simulink model "dcpController_ExperimentalPosVel"  (R2016b)
settings: Solver=ode5  StartTime=0.0  StopTime=inf  FixedStep=0.001  RelTol=1e-3  EnableMultiTasking=on
undefined symbols (not defined in the file): robot, Standard_Devices, UDP_Protocol
libraries: dcpctrl x20, simulink x6, kukaslxctrl x1, sldrtlib x1
(part 1 of 2)
settings Model: SimulationMode=external  Creator=julianleland  LastModifiedBy=julianleland
settings OptimizationCC: LifeSpan=inf
settings DebuggingCC: SFUnexpectedBacktrackingDiag=warning  SFNoUnconditionalDefaultTransitionDiag=warning  SFExecutionAtInitializationDiag=none
settings HardwareCC: ProdBitPerLong=64  ProdHWDeviceType=Intel->x86-64 (Mac OS X)  TargetBitPerLong=64  TargetBitPerPointer=64  TargetIntDivRoundTo=Zero  TargetEndianess=LittleEndian  TargetWordSize=64  TargetHWDeviceType=Intel->x86-64
settings RTWCC: SystemTargetFile=sldrt.tlc  TemplateMakefile=sldrt.tmf  Description=Simulink Desktop Real-Time  RTWCompilerOptimization=on
settings CodeAppCC: MaxIdLength=95
settings SimulinkDesktopRealTimeCC: TargetPreCompLibLocation=/Applications/MATLAB_R2016b.app/toolbox/sldrt/lib/maci64  TargetLangStandard=C89/C90 (ANSI)  SupportVariableSizeSignals=off
settings ConfigComp: CovMetricSettings=dw  CovHtmlReporting=on  CovSaveCumulativeToWorkspaceVar=on  CovSaveSingleToWorkspaceVar=on  CovExternalEMLEnable=off

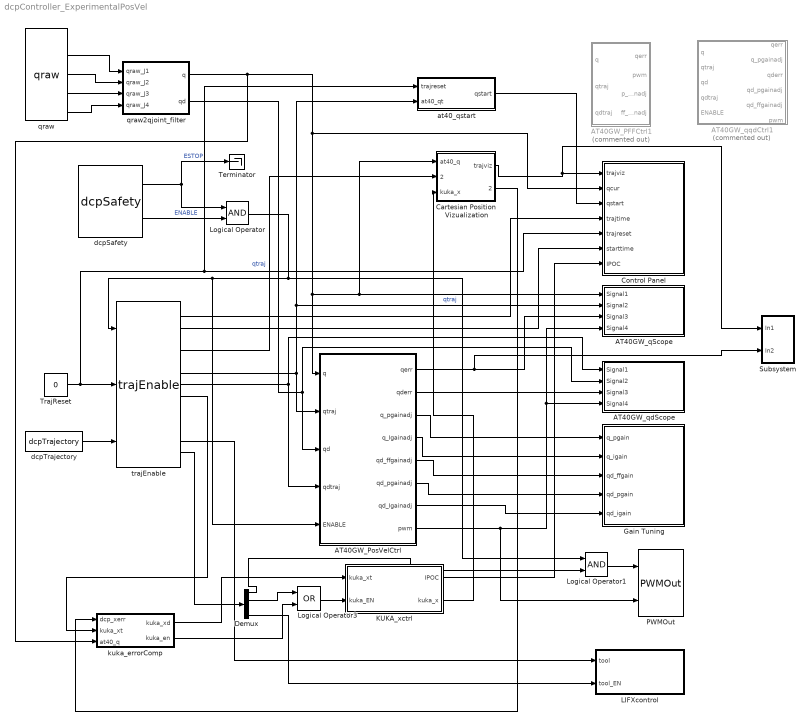
== system dcpController_ExperimentalPosVel ==
  AT40GW_PFFCtrl1 : Subsystem  Commented=on
  AT40GW_PosVelCtrl : Subsystem
  AT40GW_qScope : Subsystem  AncestorBlock=dcpctrl/AT40GW_qScope
  AT40GW_qdScope : Subsystem  AncestorBlock=dcpctrl/AT40GW_qScope
  AT40GW_qqdCtrl1 : Subsystem  Commented=on
  Cartesian Position Vizualization : Subsystem
  Control Panel : Subsystem
  Demux : Demux
  Gain Tuning : Subsystem
  KUKA_xctrl : Subsystem
  LIFXcontrol : Subsystem
  Logical Operator : Logic  AllPortsSameDT=off  OutDataTypeStr=boolean
  Logical Operator1 : Logic  AllPortsSameDT=off  OutDataTypeStr=boolean
  Logical Operator3 : Logic  Operator=OR  AllPortsSameDT=off  OutDataTypeStr=boolean
  PWMOut : dcpctrl/PWMOut
  Subsystem : Subsystem
  Terminator : Terminator
  TrajReset : Constant  Value=0
  at40_qstart : Subsystem
  dcpSafety : dcpctrl/dcpSafety
  dcpTrajectory : dcpctrl/dcpTrajectory
  kuka_errorComp : Subsystem
  qraw : dcpctrl/qraw
  qraw2qjoint_filter : Subsystem
  trajEnable : dcpctrl/trajEnable
      link override "Stoppable Time/Trajectory Time ": Gain=0
  wires:
  trajEnable/6 -> AT40GW_PosVelCtrl/2(qtraj), at40_qstart/2(at40_qt), AT40GW_qScope/2(Signal2)  "qtraj"
  dcpSafety/1 -> Logical Operator/1, Terminator/1  "ESTOP"
  dcpSafety/2 -> Logical Operator/2  "ENABLE"
  TrajReset/1 -> at40_qstart/1(trajreset), Control Panel/5(trajreset), trajEnable/2
  trajEnable/1 -> Control Panel/4(trajtime)
  qraw2qjoint_filter/1(q) -> kuka_errorComp/3(at40_q), AT40GW_PosVelCtrl/1(q), Cartesian Position Vizualization/1(at40_q), AT40GW_qScope/1(Signal1), Control Panel/2(qcur)
  trajEnable/12 -> LIFXcontrol/1(tool)
  dcpTrajectory/1 -> trajEnable/3
  trajEnable/2 -> Control Panel/6(starttime)
  qraw/2 -> qraw2qjoint_filter/1(qraw_J1)
  qraw/3 -> qraw2qjoint_filter/2(qraw_J2)
  qraw/4 -> qraw2qjoint_filter/3(qraw_J3)
  qraw/5 -> qraw2qjoint_filter/4(qraw_J4)
  Cartesian Position Vizualization/1(trajviz) -> Subsystem/1(In1), Control Panel/1(trajviz)
  KUKA_xctrl/1(IPOC) -> Control Panel/7(IPOC)
  trajEnable/8 -> kuka_errorComp/2("kuka_xt ")
  trajEnable/13 -> Demux/1
  Demux/4 -> LIFXcontrol/2(tool_EN)
  Logical Operator1/1 -> PWMOut/1
  Demux/1 -> Logical Operator1/2
  KUKA_xctrl/2(kuka_x) -> Cartesian Position Vizualization/3(kuka_x)
  trajEnable/4 -> Cartesian Position Vizualization/2(dcp_xdes)  "qtraj"
  qraw2qjoint_filter/2(qd) -> AT40GW_PosVelCtrl/3(qd), AT40GW_qdScope/2(Signal2)
  Logical Operator/1 -> Logical Operator1/1, AT40GW_PosVelCtrl/5(ENABLE), trajEnable/1
  AT40GW_PosVelCtrl/2(qderr) -> AT40GW_qdScope/3(Signal3)
  AT40GW_PosVelCtrl/8(pwm) -> AT40GW_qdScope/4(Signal4), AT40GW_qScope/4(Signal4), PWMOut/2
  trajEnable/7 -> AT40GW_qdScope/1(Signal1), AT40GW_PosVelCtrl/4(qdtraj)
  AT40GW_PosVelCtrl/1(qerr) -> Subsystem/2(In2), AT40GW_qScope/3(Signal3)
  AT40GW_PosVelCtrl/3(q_pgainadj) -> Gain Tuning/1(q_pgain)
  AT40GW_PosVelCtrl/5(qd_ffgainadj) -> Gain Tuning/3(qd_ffgain)
  AT40GW_PosVelCtrl/6(qd_pgainadj) -> Gain Tuning/4(qd_pgain)
  AT40GW_PosVelCtrl/4(q_Igainadj) -> Gain Tuning/2(q_igain)
  AT40GW_PosVelCtrl/7(qd_Igainadj) -> Gain Tuning/5(qd_igain)
  kuka_errorComp/1(kuka_xd) -> KUKA_xctrl/1("kuka_xt   ")
  Cartesian Position Vizualization/2(dcp_xerr) -> kuka_errorComp/1(dcp_xerr)
  Logical Operator3/1 -> KUKA_xctrl/2(kuka_EN)
  Demux/2 -> Logical Operator3/1
  kuka_errorComp/2(kuka_en) -> Logical Operator3/2
  at40_qstart/1(qstart) -> Control Panel/3(qstart)

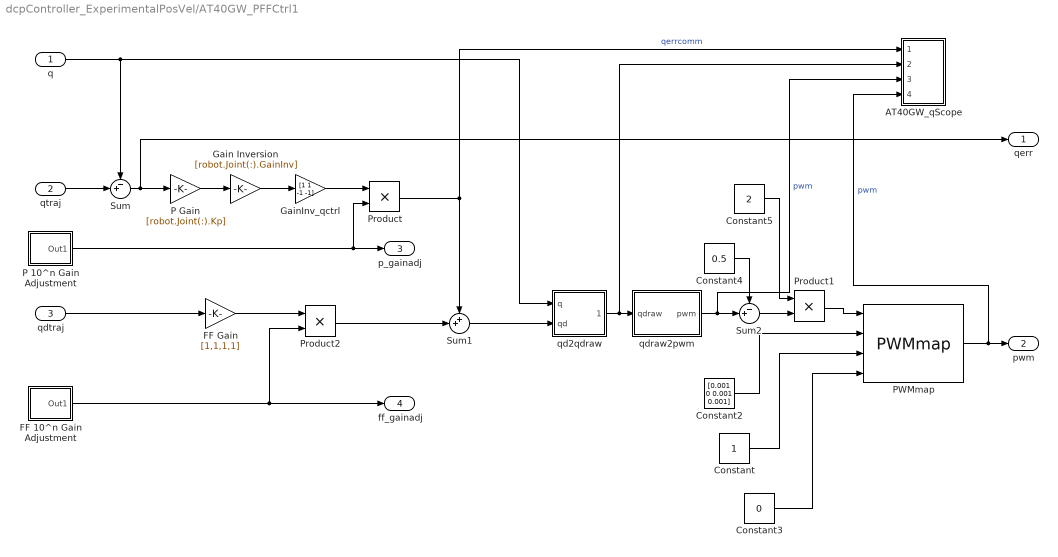
== system dcpController_ExperimentalPosVel/AT40GW_PFFCtrl1 ==
  q : Inport
  qtraj : Inport  Port=2
  qdtraj : Inport  Port=3
  AT40GW_qScope : Subsystem
  Constant : Constant
  Constant2 : Constant  Value=[0.001 0 0.001 0.001]
  Constant3 : Constant  Value=0
  Constant4 : Constant  Value=0.5
  Constant5 : Constant  Value=2
  FF 10^n Gain Adjustment : Subsystem
  FF Gain : Gain  Gain=[1,1,1,1]
  Gain Inversion : Gain  Gain=[robot.Joint(:).GainInv]
  GainInv_qctrl : Gain  Gain=[1 1 -1 -1]
  P 10^n Gain Adjustment : Subsystem
  P Gain : Gain  Gain=[robot.Joint(:).Kp]
  PWMmap : dcpctrl/PWMmap
  Product : Product
  Product1 : Product
  Product2 : Product
  Sum : Sum  Inputs=-+|
  Sum1 : Sum  Inputs=++|
  Sum2 : Sum  Inputs=-+|
  qd2qdraw : Subsystem
  qdraw2pwm : Subsystem
  qerr : Outport
  pwm : Outport  Port=2
  p_gainadj : Outport  Port=3
  ff_gainadj : Outport  Port=4
  wires:
  Product2/1 -> Sum1/2
  FF 10^n Gain Adjustment/1(Out1) -> Product2/2, ff_gainadj/1
  P 10^n Gain Adjustment/1(Out1) -> Product/2, p_gainadj/1
  Product/1 -> AT40GW_qScope/1(Signal1), Sum1/1  "qerrcomm"
  PWMmap/1 -> pwm/1, AT40GW_qScope/4(Signal4)  "pwm"
  FF Gain/1 -> Product2/1
  qdtraj/1 -> FF Gain/1
  Constant5/1 -> Product1/1
  Product1/1 -> PWMmap/1
  Sum2/1 -> Product1/2
  Constant4/1 -> Sum2/1
  qdraw2pwm/1(pwm) -> Sum2/2, AT40GW_qScope/3(Signal3)  "pwm"
  GainInv_qctrl/1 -> Product/1
  qd2qdraw/1(qdraw) -> qdraw2pwm/1(qdraw), AT40GW_qScope/2(Signal2)
  q/1 -> Sum/1, qd2qdraw/1(q)
  Sum1/1 -> qd2qdraw/2(qd)
  Gain Inversion/1 -> GainInv_qctrl/1
  Constant2/1 -> PWMmap/2
  Constant3/1 -> PWMmap/4
  Constant/1 -> PWMmap/3
  P Gain/1 -> Gain Inversion/1
  Sum/1 -> qerr/1, P Gain/1
  qtraj/1 -> Sum/2

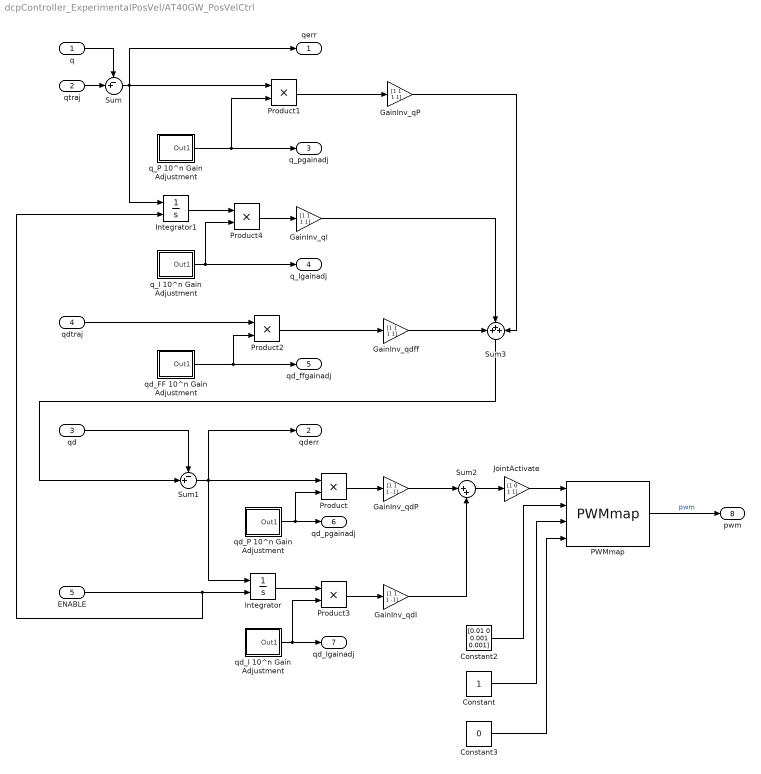
== system dcpController_ExperimentalPosVel/AT40GW_PosVelCtrl ==
  q : Inport
  qtraj : Inport  Port=2
  qd : Inport  Port=3
  qdtraj : Inport  Port=4
  ENABLE : Inport  Port=5
  Constant : Constant
  Constant2 : Constant  Value=[0.01 0 0.001 0.001]
  Constant3 : Constant  Value=0
  GainInv_qI : Gain  Gain=[1 1 1 1]
  GainInv_qP : Gain  Gain=[1 1 1 1]
  GainInv_qdI : Gain  Gain=[1 1 1 -1]
  GainInv_qdP : Gain  Gain=[1 1 1 -1]
  GainInv_qdff : Gain  Gain=[1 1 1 1]
  Integrator : Integrator  ExternalReset=rising  LimitOutput=on  UpperSaturationLimit=[100 10 100 1000]  LowerSaturationLimit=[-100 -10 -100 -1000]
  Integrator1 : Integrator  ExternalReset=rising  LimitOutput=on  UpperSaturationLimit=[10 2 10 20]  LowerSaturationLimit=[-10 -2 -10 -20]
  JointActivate : Gain  Gain=[1 0 1 1]
  PWMmap : dcpctrl/PWMmap
  Product{,1..4} (5 alike) : Product
  Sum : Sum  Inputs=-+|
  Sum1 : Sum  Inputs=-+|
  Sum2 : Sum  Inputs=|++
  Sum3 : Sum  Inputs=+++
  q_I 10^n Gain Adjustment : Subsystem
  q_P 10^n Gain Adjustment : Subsystem
  qd_FF 10^n Gain Adjustment : Subsystem
  qd_I 10^n Gain Adjustment : Subsystem
  qd_P 10^n Gain Adjustment : Subsystem
  qerr : Outport
  qderr : Outport  Port=2
  q_pgainadj : Outport  Port=3
  q_Igainadj : Outport  Port=4
  qd_ffgainadj : Outport  Port=5
  qd_pgainadj : Outport  Port=6
  qd_Igainadj : Outport  Port=7
  pwm : Outport  Port=8
  wires:
  GainInv_qdff/1 -> Sum3/1
  Sum3/1 -> Sum1/2
  GainInv_qdI/1 -> Sum2/2
  ENABLE/1 -> Integrator/2, Integrator1/2
  Integrator1/1 -> Product4/1
  Product4/1 -> GainInv_qI/1
  q_I 10^n Gain Adjustment/1(Out1) -> q_Igainadj/1, Product4/2
  Sum/1 -> Integrator1/1, qerr/1, Product1/1
  Sum2/1 -> JointActivate/1
  qdtraj/1 -> Product2/1
  qd/1 -> Sum1/1
  Integrator/1 -> Product3/1
  GainInv_qdP/1 -> Sum2/1
  Product3/1 -> GainInv_qdI/1
  qd_I 10^n Gain Adjustment/1(Out1) -> qd_Igainadj/1, Product3/2
  q_P 10^n Gain Adjustment/1(Out1) -> Product1/2, q_pgainadj/1
  Product/1 -> GainInv_qdP/1
  q/1 -> Sum/1
  Product2/1 -> GainInv_qdff/1
  Sum1/1 -> qderr/1, Product/1, Integrator/1
  qd_FF 10^n Gain Adjustment/1(Out1) -> Product2/2, qd_ffgainadj/1
  qd_P 10^n Gain Adjustment/1(Out1) -> Product/2, qd_pgainadj/1
  PWMmap/1 -> pwm/1  "pwm"
  Product1/1 -> GainInv_qP/1
  Constant2/1 -> PWMmap/2
  Constant3/1 -> PWMmap/4
  Constant/1 -> PWMmap/3
  qtraj/1 -> Sum/2
  JointActivate/1 -> PWMmap/1
  GainInv_qI/1 -> Sum3/2
  GainInv_qP/1 -> Sum3/3

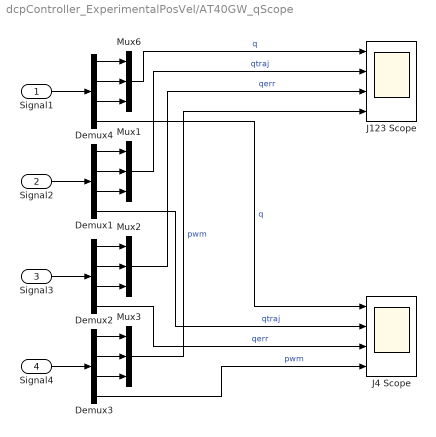
== system dcpController_ExperimentalPosVel/AT40GW_qScope ==
  Signal1 : Inport
  Signal2 : Inport  Port=2
  Signal3 : Inport  Port=3
  Signal4 : Inport  Port=4
  Demux{1..4} (4 alike) : Demux
  J123 Scope : Scope  NumInputPorts=4
  J4 Scope : Scope  NumInputPorts=4
  Mux{1..3,6} (4 alike) : Mux  Inputs=3
  wires:
  Demux4/1 -> Mux6/1
  Mux3/1 -> J123 Scope/4  "pwm"
  Demux2/4 -> J4 Scope/3  "qerr"
  Demux1/4 -> J4 Scope/2  "qtraj"
  Mux6/1 -> J123 Scope/1  "q"
  Signal1/1 -> Demux4/1
  Demux4/2 -> Mux6/2
  Demux4/3 -> Mux6/3
  Demux1/1 -> Mux1/1
  Signal2/1 -> Demux1/1
  Demux1/2 -> Mux1/2
  Demux1/3 -> Mux1/3
  Demux2/1 -> Mux2/1
  Signal3/1 -> Demux2/1
  Demux2/2 -> Mux2/2
  Demux2/3 -> Mux2/3
  Demux3/1 -> Mux3/1
  Signal4/1 -> Demux3/1
  Demux3/2 -> Mux3/2
  Demux3/3 -> Mux3/3
  Mux1/1 -> J123 Scope/2  "qtraj"
  Mux2/1 -> J123 Scope/3  "qerr"
  Demux4/4 -> J4 Scope/1  "q"
  Demux3/4 -> J4 Scope/4  "pwm"

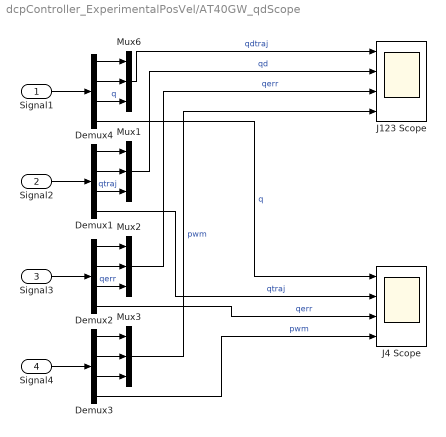
== system dcpController_ExperimentalPosVel/AT40GW_qdScope ==
  Signal1 : Inport
  Signal2 : Inport  Port=2
  Signal3 : Inport  Port=3
  Signal4 : Inport  Port=4
  Demux{1..4} (4 alike) : Demux
  J123 Scope : Scope  NumInputPorts=4
  J4 Scope : Scope  NumInputPorts=4
  Mux{1..3,6} (4 alike) : Mux  Inputs=3
  wires:
  Demux3/4 -> J4 Scope/4  "pwm"
  Demux4/4 -> J4 Scope/1  "q"
  Demux2/3 -> Mux2/3  "qerr"
  Demux1/3 -> Mux1/3  "qtraj"
  Demux3/3 -> Mux3/3
  Demux3/2 -> Mux3/2
  Signal4/1 -> Demux3/1
  Demux3/1 -> Mux3/1
  Demux2/2 -> Mux2/2
  Signal3/1 -> Demux2/1
  Demux2/1 -> Mux2/1
  Demux1/2 -> Mux1/2
  Signal2/1 -> Demux1/1
  Demux1/1 -> Mux1/1
  Signal1/1 -> Demux4/1
  Demux4/3 -> Mux6/3  "q"
  Demux1/4 -> J4 Scope/2  "qtraj"
  Demux2/4 -> J4 Scope/3  "qerr"
  Mux3/1 -> J123 Scope/4  "pwm"
  Demux4/1 -> Mux6/1
  Demux4/2 -> Mux6/2
  Mux6/1 -> J123 Scope/1  "qdtraj"
  Mux1/1 -> J123 Scope/2  "qd"
  Mux2/1 -> J123 Scope/3  "qerr"

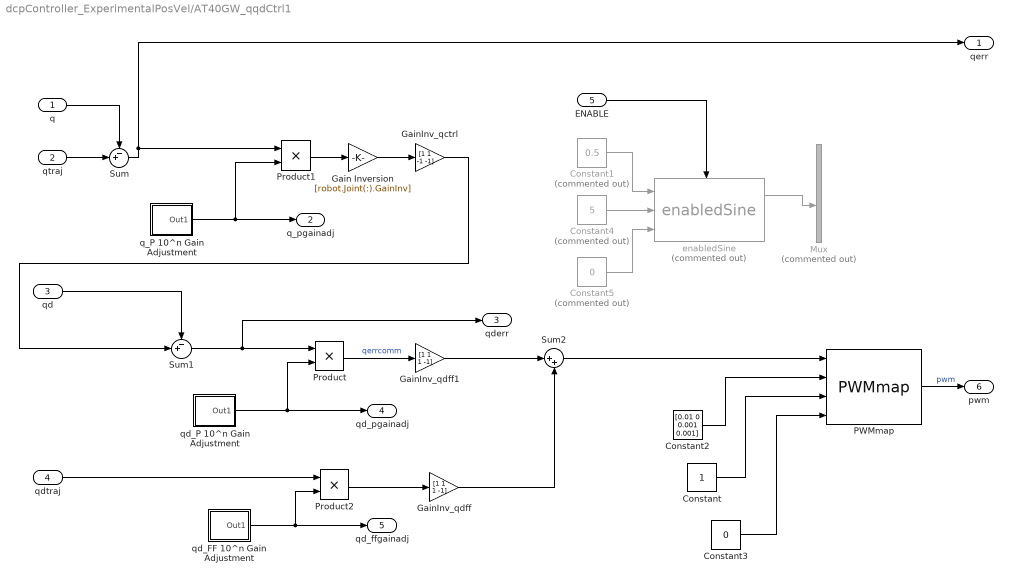
== system dcpController_ExperimentalPosVel/AT40GW_qqdCtrl1 ==
  q : Inport
  qtraj : Inport  Port=2
  qd : Inport  Port=3
  qdtraj : Inport  Port=4
  ENABLE : Inport  Port=5
  Constant : Constant
  Constant1 : Constant  Commented=on  Value=0.5
  Constant2 : Constant  Value=[0.01 0 0.001 0.001]
  Constant3 : Constant  Value=0
  Constant4 : Constant  Commented=on  Value=5
  Constant5 : Constant  Commented=on  Value=0
  Gain Inversion : Gain  Gain=[robot.Joint(:).GainInv]
  GainInv_qctrl : Gain  Gain=[1 1 -1 -1]
  GainInv_qdff : Gain  Gain=[1 1 1 -1]
  GainInv_qdff1 : Gain  Gain=[1 1 1 -1]
  Mux : Mux  Commented=on
  PWMmap : dcpctrl/PWMmap
  Product : Product
  Product1 : Product
  Product2 : Product
  Sum : Sum  Inputs=-+|
  Sum1 : Sum  Inputs=-+|
  Sum2 : Sum  Inputs=|++
  enabledSine : dcpctrl/enabledSine  Commented=on
  q_P 10^n Gain Adjustment : Subsystem
  qd_FF 10^n Gain Adjustment : Subsystem
  qd_P 10^n Gain Adjustment : Subsystem
  qerr : Outport
  q_pgainadj : Outport  Port=2
  qderr : Outport  Port=3
  qd_pgainadj : Outport  Port=4
  qd_ffgainadj : Outport  Port=5
  pwm : Outport  Port=6
  wires:
  GainInv_qctrl/1 -> Sum1/2
  q_P 10^n Gain Adjustment/1(Out1) -> Product1/2, q_pgainadj/1
  GainInv_qdff/1 -> Sum2/2
  Constant5/1 -> enabledSine/3
  Constant4/1 -> enabledSine/2
  Constant1/1 -> enabledSine/1
  ENABLE/1 -> enabledSine/Enable
  enabledSine/1 -> Mux/3
  Sum2/1 -> PWMmap/1
  GainInv_qdff1/1 -> Sum2/1
  Product/1 -> GainInv_qdff1/1  "qerrcomm"
  q/1 -> Sum/1
  Product2/1 -> GainInv_qdff/1
  Sum1/1 -> qderr/1, Product/1
  qdtraj/1 -> Product2/1
  qd/1 -> Sum1/1
  qd_FF 10^n Gain Adjustment/1(Out1) -> Product2/2, qd_ffgainadj/1
  qd_P 10^n Gain Adjustment/1(Out1) -> Product/2, qd_pgainadj/1
  PWMmap/1 -> pwm/1  "pwm"
  Gain Inversion/1 -> GainInv_qctrl/1
  Constant2/1 -> PWMmap/2
  Constant3/1 -> PWMmap/4
  Constant/1 -> PWMmap/3
  Product1/1 -> Gain Inversion/1
  Sum/1 -> qerr/1, Product1/1
  qtraj/1 -> Sum/2

== system dcpController_ExperimentalPosVel/Cartesian Position Vizualization ==
  at40_q : Inport
  dcp_xdes : Inport  Port=2
  kuka_x : Inport  Port=3
  Mux : Mux  Inputs=2
  Sum : Sum
  Sum1 : Sum  Inputs=+-
  fkine_at40gw : MATLAB Function  TreatAsAtomicUnit=on
  trajviz : Outport
  dcp_xerr : Outport  Port=2
  wires:
  at40_q/1 -> fkine_at40gw/1(q)
  fkine_at40gw/1(x) -> Sum1/1, Sum/2
  Mux/1 -> trajviz/1
  Sum/1 -> Mux/1
  kuka_x/1 -> Sum/1
  dcp_xdes/1 -> Sum1/2, Mux/2
  Sum1/1 -> dcp_xerr/1

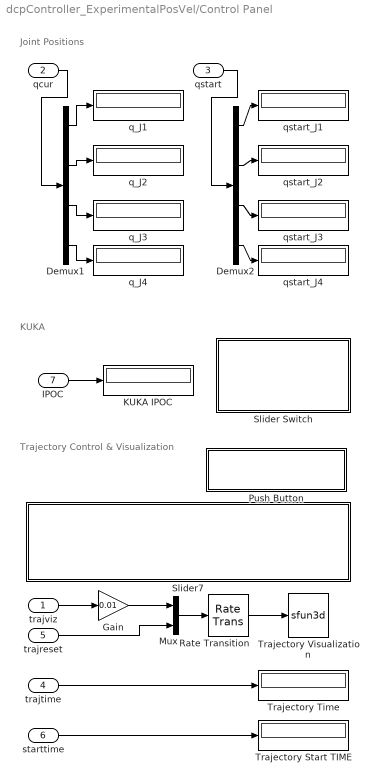
== system dcpController_ExperimentalPosVel/Control Panel ==
  note: KUKA
  note: Joint Positions
  note: Trajectory Control & Visualization
  trajviz : Inport
  qcur : Inport  Port=2
  qstart : Inport  Port=3
  trajtime : Inport  Port=4
  trajreset : Inport  Port=5
  starttime : Inport  Port=6
  IPOC : Inport  Port=7
  Demux1 : Demux
  Demux2 : Demux
  Gain : Gain  Gain=0.01
  KUKA IPOC : Display
  Mux : Mux  Inputs=2
  Push Button : Subsystem  DialogController=hmiCreateDDGDialog  IsWebBlock=on  mask(MWDashboardBlock){webBlockId=d14440dc-dcfb-4a22-9820-9883405fda4f, webBlockType=pushbutton, ShowInLibBrwoser=on, ShowInitialText=on, HMISrcModelName=dcpController_ExperimentalPosVel}
      mask prompts: webBlockId "WebBlock Id"; webBlockType "WebBlock Type"; HMISrcModelName "Source Model"
      mask Help: helpview([docroot '/mapfiles/simulink.map'], 'hmi_push_button')
      mask Display:
      | model = bdroot(gcb);
      | if strcmp(get_param(model,'BlockDiagramType'), 'library')
      |     image([(matlabroot) '/toolbox/simulink/hmi/icons/PushButton.png']);
      | end
  Rate Transition : RateTransition
  Slider Switch : Subsystem  DialogController=hmiCreateDDGDialog  IsWebBlock=on  mask(MWDashboardBlock){webBlockId=b2d97664-68dd-4dea-8ae4-c535c985ddf0, webBlockType=sliderswitch, ShowInLibBrowser=on, ShowInitialText=on, HMISrcModelName=dcpController_ExperimentalPosVel}
      mask prompts: webBlockId "WebBlock Id"; webBlockType "WebBlock Type"; HMISrcModelName "Source Model"
      mask help: SimulinkHMI:dialogs:SwitchDialogDesc
      mask Help: helpview([docroot '/mapfiles/simulink.map'], 'hmi_slider_switch')
      mask Display:
      | if strcmp(get_param(bdroot(gcb),'BlockDiagramType'), 'library')
      |     image([(matlabroot) '/toolbox/simulink/hmi/icons/SliderSwitch.png']);
      | end
  Slider7 : Subsystem  DialogController=hmiCreateDDGDialog  IsWebBlock=on  mask(MWDashboardBlock){webBlockId=8192e4e1-ec01-457d-8e28-0b86459142e6, webBlockType=slider, ShowInLibBrowser=on, ShowInitialText=on, HMISrcModelName=dcpController_ExperimentalPosVel}
      mask prompts: webBlockId "WebBlock Id"; webBlockType "WebBlock Type"; HMISrcModelName "Source Model"
      mask Help: helpview([docroot '/mapfiles/simulink.map'], 'hmi_slider')
      mask Display:
      | if strcmp(get_param(bdroot(gcb),'BlockDiagramType'), 'library')
      |     image([(matlabroot) '/toolbox/simulink/hmi/icons/Slider.png']);
      | end
  Trajectory Visualization : S-Function  LoadFcn=if exist('sfun3d','file'), sfun3d([],[],[],'LoadBlock'); end  FunctionName=sfun3d  Parameters=ax,T,np,cp,gd,ls,mk  SFunctionDeploymentMode=off  EnableBusSupport=off  mask(3D Graph){np=2, ax=[30 80 -20 20 -10 30], cp=[80 10 20], gd=on, ls=-, mk=., T=0.1}
      mask prompts: np "Number of point (lines)"; ax "[xmin xmax  ymin ymax zmin zmax]"; cp "Camera position (use [0 0 1] for 2D XY view)"; gd "Grid (on|off)"; ls "LineStyle"; mk "Marker"; T "Sampling Time"
      mask help:
      | This block plots the position of several points in the XYZ space. The input contains the coordinates of all the points (x1,y1,z1,x2,y2,z2,...).
      | The number of points (lines), the XYZ ranges, camera position, grid, linestyle, marker and sampling time, can be set as mask parameters.
      settings: CopyFcn=if exist('sfun3d','file'), sfun3d([],[],[],'CopyBlock'); end  DeleteFcn=if exist('sfun3d','file'), sfun3d([],[],[],'DeleteBlock'); end  NameChangeFcn=if exist('sfun3d','file'), sfun3d([],[],[],'NameChange'); end
      mask Help:
      | This block plots the position of several points in the XYZ space. The input contains the coordinates of all the points (x1,y1,z1,x2,y2,z2,...).
      | The number of points (lines), the XYZ ranges, camera position, grid, linestyle, marker and sampling time, can be set as mask parameters.
      mask TypeOptions ls: - | -- | : | -. | none
      mask TypeOptions mk: none | . | + | o | * | x | square | diamond | v | ^ | > | < | pentagram | hexagram
      mask Display: plot([.05 .95 .95 .05 .05],[.45 .45 .95 .95 .45], 0.5+cos(0:0.1:2*pi)*0.3,0.7+sin(0:0.1:2*pi)*0.2)
  Trajectory Start TIME : Display
  Trajectory Time : Display
  q_J{1..4} (4 alike) : Display
  qstart_J{1..4} (4 alike) : Display
  wires:
  qcur/1 -> Demux1/1
  Demux1/4 -> q_J4/1
  Demux1/1 -> q_J1/1
  Demux1/3 -> q_J3/1
  Demux1/2 -> q_J2/1
  qstart/1 -> Demux2/1
  Demux2/4 -> qstart_J4/1
  Demux2/1 -> qstart_J1/1
  Demux2/3 -> qstart_J3/1
  Demux2/2 -> qstart_J2/1
  trajtime/1 -> Trajectory Time/1
  trajviz/1 -> Gain/1
  Gain/1 -> Mux/1
  Mux/1 -> Rate Transition/1
  Rate Transition/1 -> Trajectory Visualization/1
  trajreset/1 -> Mux/2
  starttime/1 -> Trajectory Start TIME/1
  IPOC/1 -> KUKA IPOC/1

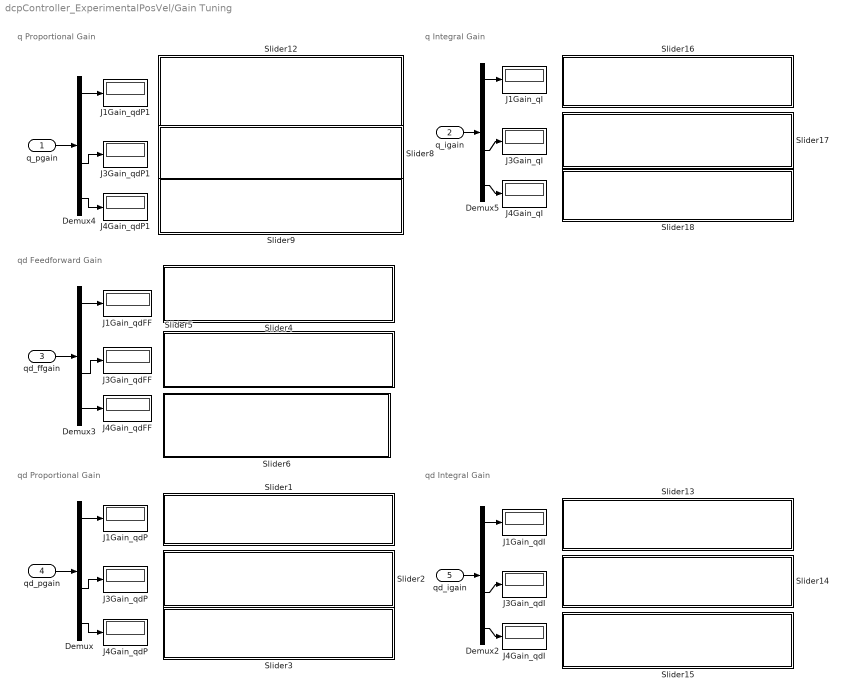
== system dcpController_ExperimentalPosVel/Gain Tuning ==
  note: q Integral Gain
  note: q Proportional Gain
  note: qd Proportional Gain
  note: qd Feedforward Gain
  note: qd Integral Gain
  q_pgain : Inport
  q_igain : Inport  Port=2
  qd_ffgain : Inport  Port=3
  qd_pgain : Inport  Port=4
  qd_igain : Inport  Port=5
  Demux{,2..5} (5 alike) : Demux
  J1Gain_qI : Display
  J1Gain_qdFF : Display
  J1Gain_qdI : Display
  J1Gain_qdP : Display
  J1Gain_qdP1 : Display
  J3Gain_qI : Display
  J3Gain_qdFF : Display
  J3Gain_qdI : Display
  J3Gain_qdP : Display
  J3Gain_qdP1 : Display
  J4Gain_qI : Display
  J4Gain_qdFF : Display
  J4Gain_qdI : Display
  J4Gain_qdP : Display
  J4Gain_qdP1 : Display
  Slider1 : Subsystem  DialogController=hmiCreateDDGDialog  IsWebBlock=on  mask(MWDashboardBlock){webBlockId=3c50ff6e-68c9-4e29-bc5d-27fb2c1dd185, webBlockType=slider, ShowInLibBrowser=on, ShowInitialText=on, HMISrcModelName=dcpController_ExperimentalPosVel}
      mask prompts: webBlockId "WebBlock Id"; webBlockType "WebBlock Type"; HMISrcModelName "Source Model"
      mask Help: helpview([docroot '/mapfiles/simulink.map'], 'hmi_slider')
      mask Display:
      | if strcmp(get_param(bdroot(gcb),'BlockDiagramType'), 'library')
      |     image([(matlabroot) '/toolbox/simulink/hmi/icons/Slider.png']);
      | end
  Slider12 : Subsystem  DialogController=hmiCreateDDGDialog  IsWebBlock=on  mask(MWDashboardBlock){webBlockId=98d1e80e-13d0-480f-8552-968791046da6, webBlockType=slider, ShowInLibBrowser=on, ShowInitialText=on, HMISrcModelName=dcpController_ExperimentalPosVel}
      mask prompts: webBlockId "WebBlock Id"; webBlockType "WebBlock Type"; HMISrcModelName "Source Model"
      mask help: SimulinkHMI:dialogs:SliderDialogDesc
      mask Help: helpview([docroot '/mapfiles/simulink.map'], 'hmi_slider')
      mask Display:
      | if strcmp(get_param(bdroot(gcb),'BlockDiagramType'), 'library')
      |     image([(matlabroot) '/toolbox/simulink/hmi/icons/Slider.png']);
      | end
  Slider13 : Subsystem  DialogController=hmiCreateDDGDialog  IsWebBlock=on  mask(MWDashboardBlock){webBlockId=6500f09a-ba96-4932-a722-58cf661d40e0, webBlockType=slider, ShowInLibBrowser=on, ShowInitialText=on, HMISrcModelName=dcpController_ExperimentalPosVel}
      mask prompts: webBlockId "WebBlock Id"; webBlockType "WebBlock Type"; HMISrcModelName "Source Model"
      mask Help: helpview([docroot '/mapfiles/simulink.map'], 'hmi_slider')
      mask Display:
      | if strcmp(get_param(bdroot(gcb),'BlockDiagramType'), 'library')
      |     image([(matlabroot) '/toolbox/simulink/hmi/icons/Slider.png']);
      | end
  Slider14 : Subsystem  DialogController=hmiCreateDDGDialog  IsWebBlock=on  mask(MWDashboardBlock){webBlockId=ae3c1573-e4c4-40ad-931a-a07230b1b4b6, webBlockType=slider, ShowInLibBrowser=on, ShowInitialText=on, HMISrcModelName=dcpController_ExperimentalPosVel}
      mask prompts: webBlockId "WebBlock Id"; webBlockType "WebBlock Type"; HMISrcModelName "Source Model"
      mask Help: helpview([docroot '/mapfiles/simulink.map'], 'hmi_slider')
      mask Display:
      | if strcmp(get_param(bdroot(gcb),'BlockDiagramType'), 'library')
      |     image([(matlabroot) '/toolbox/simulink/hmi/icons/Slider.png']);
      | end
  Slider15 : Subsystem  DialogController=hmiCreateDDGDialog  IsWebBlock=on  mask(MWDashboardBlock){webBlockId=4d11668a-e4ea-4c4b-be96-35fa626a327f, webBlockType=slider, ShowInLibBrowser=on, ShowInitialText=on, HMISrcModelName=dcpController_ExperimentalPosVel}
      mask prompts: webBlockId "WebBlock Id"; webBlockType "WebBlock Type"; HMISrcModelName "Source Model"
      mask Help: helpview([docroot '/mapfiles/simulink.map'], 'hmi_slider')
      mask Display:
      | if strcmp(get_param(bdroot(gcb),'BlockDiagramType'), 'library')
      |     image([(matlabroot) '/toolbox/simulink/hmi/icons/Slider.png']);
      | end
  Slider16 : Subsystem  DialogController=hmiCreateDDGDialog  IsWebBlock=on  mask(MWDashboardBlock){webBlockId=504a68a0-da33-45da-aa03-381331d012b0, webBlockType=slider, ShowInLibBrowser=on, ShowInitialText=on, HMISrcModelName=dcpController_ExperimentalPosVel}
      mask prompts: webBlockId "WebBlock Id"; webBlockType "WebBlock Type"; HMISrcModelName "Source Model"
      mask Help: helpview([docroot '/mapfiles/simulink.map'], 'hmi_slider')
      mask Display:
      | if strcmp(get_param(bdroot(gcb),'BlockDiagramType'), 'library')
      |     image([(matlabroot) '/toolbox/simulink/hmi/icons/Slider.png']);
      | end
  Slider17 : Subsystem  DialogController=hmiCreateDDGDialog  IsWebBlock=on  mask(MWDashboardBlock){webBlockId=7bbe7755-d2df-42f7-a1c1-4b4527655fe8, webBlockType=slider, ShowInLibBrowser=on, ShowInitialText=on, HMISrcModelName=dcpController_ExperimentalPosVel}
      mask prompts: webBlockId "WebBlock Id"; webBlockType "WebBlock Type"; HMISrcModelName "Source Model"
      mask Help: helpview([docroot '/mapfiles/simulink.map'], 'hmi_slider')
      mask Display:
      | if strcmp(get_param(bdroot(gcb),'BlockDiagramType'), 'library')
      |     image([(matlabroot) '/toolbox/simulink/hmi/icons/Slider.png']);
      | end
  Slider18 : Subsystem  DialogController=hmiCreateDDGDialog  IsWebBlock=on  mask(MWDashboardBlock){webBlockId=2d93fa1e-30ce-4b2a-b1ce-a25975403945, webBlockType=slider, ShowInLibBrowser=on, ShowInitialText=on, HMISrcModelName=dcpController_ExperimentalPosVel}
      mask prompts: webBlockId "WebBlock Id"; webBlockType "WebBlock Type"; HMISrcModelName "Source Model"
      mask Help: helpview([docroot '/mapfiles/simulink.map'], 'hmi_slider')
      mask Display:
      | if strcmp(get_param(bdroot(gcb),'BlockDiagramType'), 'library')
      |     image([(matlabroot) '/toolbox/simulink/hmi/icons/Slider.png']);
      | end
  Slider2 : Subsystem  DialogController=hmiCreateDDGDialog  IsWebBlock=on  mask(MWDashboardBlock){webBlockId=9ee13952-8d79-48b0-b443-0ea8f888d721, webBlockType=slider, ShowInLibBrowser=on, ShowInitialText=on, HMISrcModelName=dcpController_ExperimentalPosVel}
      mask prompts: webBlockId "WebBlock Id"; webBlockType "WebBlock Type"; HMISrcModelName "Source Model"
      mask Help: helpview([docroot '/mapfiles/simulink.map'], 'hmi_slider')
      mask Display:
      | if strcmp(get_param(bdroot(gcb),'BlockDiagramType'), 'library')
      |     image([(matlabroot) '/toolbox/simulink/hmi/icons/Slider.png']);
      | end
  Slider3 : Subsystem  DialogController=hmiCreateDDGDialog  IsWebBlock=on  mask(MWDashboardBlock){webBlockId=0bbb50e3-7e9f-40d4-ad9a-fe9f4a38d1d4, webBlockType=slider, ShowInLibBrowser=on, ShowInitialText=on, HMISrcModelName=dcpController_ExperimentalPosVel}
      mask prompts: webBlockId "WebBlock Id"; webBlockType "WebBlock Type"; HMISrcModelName "Source Model"
      mask Help: helpview([docroot '/mapfiles/simulink.map'], 'hmi_slider')
      mask Display:
      | if strcmp(get_param(bdroot(gcb),'BlockDiagramType'), 'library')
      |     image([(matlabroot) '/toolbox/simulink/hmi/icons/Slider.png']);
      | end
  Slider4 : Subsystem  DialogController=hmiCreateDDGDialog  IsWebBlock=on  mask(MWDashboardBlock){webBlockId=3d64281d-80ee-431f-9059-8c619ac44f3c, webBlockType=slider, ShowInLibBrowser=on, ShowInitialText=on, HMISrcModelName=dcpController_ExperimentalPosVel}
      mask prompts: webBlockId "WebBlock Id"; webBlockType "WebBlock Type"; HMISrcModelName "Source Model"
      mask Help: helpview([docroot '/mapfiles/simulink.map'], 'hmi_slider')
      mask Display:
      | if strcmp(get_param(bdroot(gcb),'BlockDiagramType'), 'library')
      |     image([(matlabroot) '/toolbox/simulink/hmi/icons/Slider.png']);
      | end
  Slider5 : Subsystem  DialogController=hmiCreateDDGDialog  IsWebBlock=on  mask(MWDashboardBlock){webBlockId=2a644570-58ea-4010-b8bb-7a2a9bb5cf2d, webBlockType=slider, ShowInLibBrowser=on, ShowInitialText=on, HMISrcModelName=dcpController_ExperimentalPosVel}
      mask prompts: webBlockId "WebBlock Id"; webBlockType "WebBlock Type"; HMISrcModelName "Source Model"
      mask Help: helpview([docroot '/mapfiles/simulink.map'], 'hmi_slider')
      mask Display:
      | if strcmp(get_param(bdroot(gcb),'BlockDiagramType'), 'library')
      |     image([(matlabroot) '/toolbox/simulink/hmi/icons/Slider.png']);
      | end
  Slider6 : Subsystem  DialogController=hmiCreateDDGDialog  IsWebBlock=on  mask(MWDashboardBlock){webBlockId=9265b818-0918-4d39-82cc-9c0d8e2c66c5, webBlockType=slider, ShowInLibBrowser=on, ShowInitialText=on, HMISrcModelName=dcpController_ExperimentalPosVel}
      mask prompts: webBlockId "WebBlock Id"; webBlockType "WebBlock Type"; HMISrcModelName "Source Model"
      mask Help: helpview([docroot '/mapfiles/simulink.map'], 'hmi_slider')
      mask Display:
      | if strcmp(get_param(bdroot(gcb),'BlockDiagramType'), 'library')
      |     image([(matlabroot) '/toolbox/simulink/hmi/icons/Slider.png']);
      | end
  Slider8 : Subsystem  DialogController=hmiCreateDDGDialog  IsWebBlock=on  mask(MWDashboardBlock){webBlockId=3f7a891a-a27e-4d11-bc63-2d89818bf210, webBlockType=slider, ShowInLibBrowser=on, ShowInitialText=on, HMISrcModelName=dcpController_ExperimentalPosVel}
      mask prompts: webBlockId "WebBlock Id"; webBlockType "WebBlock Type"; HMISrcModelName "Source Model"
      mask help: SimulinkHMI:dialogs:SliderDialogDesc
      mask Help: helpview([docroot '/mapfiles/simulink.map'], 'hmi_slider')
      mask Display:
      | if strcmp(get_param(bdroot(gcb),'BlockDiagramType'), 'library')
      |     image([(matlabroot) '/toolbox/simulink/hmi/icons/Slider.png']);
      | end
  Slider9 : Subsystem  DialogController=hmiCreateDDGDialog  IsWebBlock=on  mask(MWDashboardBlock){webBlockId=209a5fc0-aa21-4327-87e8-0feb9346f2d8, webBlockType=slider, ShowInLibBrowser=on, ShowInitialText=on, HMISrcModelName=dcpController_ExperimentalPosVel}
      mask prompts: webBlockId "WebBlock Id"; webBlockType "WebBlock Type"; HMISrcModelName "Source Model"
      mask help: SimulinkHMI:dialogs:SliderDialogDesc
      mask Help: helpview([docroot '/mapfiles/simulink.map'], 'hmi_slider')
      mask Display:
      | if strcmp(get_param(bdroot(gcb),'BlockDiagramType'), 'library')
      |     image([(matlabroot) '/toolbox/simulink/hmi/icons/Slider.png']);
      | end
  wires:
  Demux5/3 -> J3Gain_qI/1
  Demux5/1 -> J1Gain_qI/1
  Demux5/4 -> J4Gain_qI/1
  q_igain/1 -> Demux5/1
  Demux2/3 -> J3Gain_qdI/1
  Demux2/1 -> J1Gain_qdI/1
  Demux2/4 -> J4Gain_qdI/1
  qd_igain/1 -> Demux2/1
  Demux4/3 -> J3Gain_qdP1/1
  Demux4/1 -> J1Gain_qdP1/1
  Demux4/4 -> J4Gain_qdP1/1
  q_pgain/1 -> Demux4/1
  Demux3/3 -> J3Gain_qdFF/1
  Demux3/1 -> J1Gain_qdFF/1
  Demux3/4 -> J4Gain_qdFF/1
  qd_ffgain/1 -> Demux3/1
  Demux/3 -> J3Gain_qdP/1
  Demux/1 -> J1Gain_qdP/1
  Demux/4 -> J4Gain_qdP/1
  qd_pgain/1 -> Demux/1

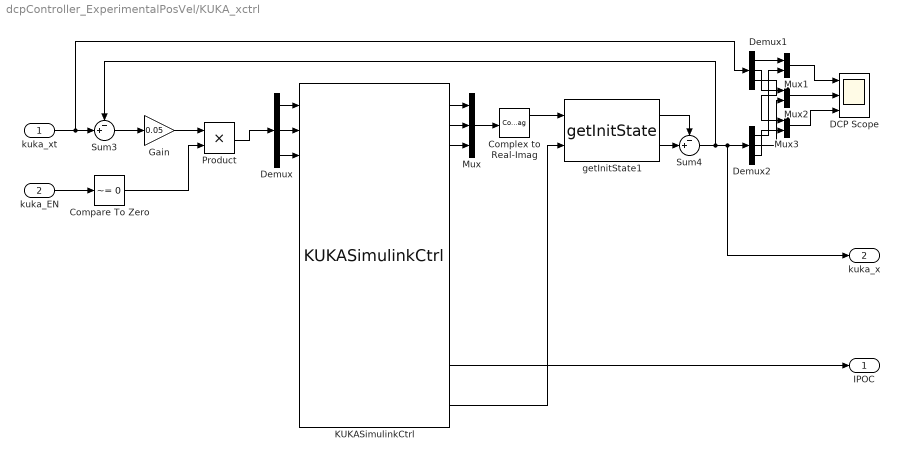
== system dcpController_ExperimentalPosVel/KUKA_xctrl ==
  "kuka_xt   " : Inport
  kuka_EN : Inport  Port=2
  Compare To Zero : simulink/Logic and Bit Operations/Compare To Zero  relop=~=  OutDataTypeStr=boolean
  Complex to Real-Imag : ComplexToRealImag
  DCP Scope : Scope  NumInputPorts=3
  Demux : Demux  Outputs=3
  Demux1 : Demux  Outputs=3
  Demux2 : Demux  Outputs=3
  Gain : Gain  Gain=0.05
  KUKASimulinkCtrl : kukaslxctrl/KUKASimulinkCtrl
  Mux : Mux  Inputs=3
  Mux1 : Mux  Inputs=2
  Mux2 : Mux  Inputs=2
  Mux3 : Mux  Inputs=2
  Product : Product
  Sum3 : Sum  Inputs=-+|
  Sum4 : Sum  Inputs=-+|
  getInitState1 : dcpctrl/getInitState
  IPOC : Outport
  kuka_x : Outport  Port=2
  wires:
  KUKASimulinkCtrl/16 -> getInitState1/2
  KUKASimulinkCtrl/2 -> Mux/2
  Sum4/1 -> kuka_x/1, Demux2/1, Sum3/1
  KUKASimulinkCtrl/14 -> IPOC/1
  KUKASimulinkCtrl/1 -> Mux/1
  Complex to Real-Imag/1 -> getInitState1/1
  KUKASimulinkCtrl/3 -> Mux/3
  Demux/2 -> KUKASimulinkCtrl/2
  Demux/3 -> KUKASimulinkCtrl/3
  Mux/1 -> Complex to Real-Imag/1
  getInitState1/1 -> Sum4/1
  getInitState1/2 -> Sum4/2
  Demux/1 -> KUKASimulinkCtrl/1
  Demux1/1 -> Mux1/1
  Mux1/1 -> DCP Scope/1
  Demux2/1 -> Mux1/2
  Mux2/1 -> DCP Scope/2
  Demux1/2 -> Mux2/1
  Mux3/1 -> DCP Scope/3
  Demux2/3 -> Mux3/2
  Demux2/2 -> Mux2/2
  Demux1/3 -> Mux3/1
  "kuka_xt   "/1 -> Sum3/2, Demux1/1
  Sum3/1 -> Gain/1
  kuka_EN/1 -> Compare To Zero/1
  Gain/1 -> Product/1
  Product/1 -> Demux/1
  Compare To Zero/1 -> Product/2

== system dcpController_ExperimentalPosVel/LIFXcontrol ==
  tool : Inport
  tool_EN : Inport  Port=2
  Compare To Zero : simulink/Logic and Bit Operations/Compare To Zero  relop=~=  OutDataTypeStr=boolean
  Constant3 : Constant  Value=3500  OutMin=[2500]  OutMax=[9000]  OutDataTypeStr=double
  Demux : Demux  Outputs=6
  Gain : Gain  Gain=360
  Hue Changer : MATLAB Function  TreatAsAtomicUnit=on
  Product : Product
  Rate Transition : RateTransition
  Rounding Function : Rounding  Operator=round
  Stream Output : sldrtlib/Stream Output  SampleTime=.1  MaxMissedTicks=10  ShowMissedTicks=off  YieldWhenWaiting=on  DrvName=Standard_Devices/UDP_Protocol  DrvAddress=54359  DrvOptions=[174338150 56700]  PortSizes=49  FormatString=repmat('%c',1,49)  ShowReady=off  ShowError=off  InitialValue=[]  FinalValue=[]
      settings: AttributesFormatString=Standard Devices\nUDP Protocol [D457h]
  qstart_J4 : Display
  wires:
  Hue Changer/1(y) -> Rate Transition/1
  Demux/2 -> Hue Changer/2(s)
  Constant3/1 -> Hue Changer/4(k)
  Rounding Function/1 -> Hue Changer/1(h), qstart_J4/1
  tool/1 -> Demux/1
  Rate Transition/1 -> Stream Output/1
  Demux/1 -> Gain/1
  Gain/1 -> Rounding Function/1
  tool_EN/1 -> Compare To Zero/1
  Compare To Zero/1 -> Product/2
  Demux/3 -> Product/1
  Product/1 -> Hue Changer/3(b)

== system dcpController_ExperimentalPosVel/Subsystem ==
  In1 : Inport
  In2 : Inport  Port=2
  DCP Scope : Scope  NumInputPorts=5
  Demux1 : Demux  Outputs=6
  Demux2 : Demux
  Mux : Mux  Inputs=3
  Mux1 : Mux  Inputs=3
  Sum : Sum  Inputs=|+-
  wires:
  Demux2/1 -> DCP Scope/3
  Demux1/1 -> Mux/1
  Demux1/5 -> Mux1/2
  Demux2/4 -> DCP Scope/5
  In2/1 -> Demux2/1
  Demux1/2 -> Mux/2
  In1/1 -> Demux1/1
  Demux1/3 -> Mux/3
  Mux/1 -> Sum/1, DCP Scope/1
  Demux1/6 -> Mux1/3
  Demux2/3 -> DCP Scope/4
  Demux1/4 -> Mux1/1
  Mux1/1 -> Sum/2
  Sum/1 -> DCP Scope/2

== system dcpController_ExperimentalPosVel/at40_qstart ==
  trajreset : Inport
  at40_qt : Inport  Port=2
  Logical Operator2 : Logic  Operator=OR  AllPortsSameDT=off  OutDataTypeStr=boolean
  Step : Step  Time=0  SampleTime=0
  Step1 : Step  Time=0.1  After=-1  SampleTime=0
  Sum : Sum  Inputs=|++
  getInitState : dcpctrl/getInitState
  qstart : Outport
  wires:
  Logical Operator2/1 -> getInitState/2
  Step/1 -> Sum/1
  at40_qt/1 -> getInitState/1
  trajreset/1 -> Logical Operator2/2
  getInitState/1 -> qstart/1
  Step1/1 -> Sum/2
  Sum/1 -> Logical Operator2/1

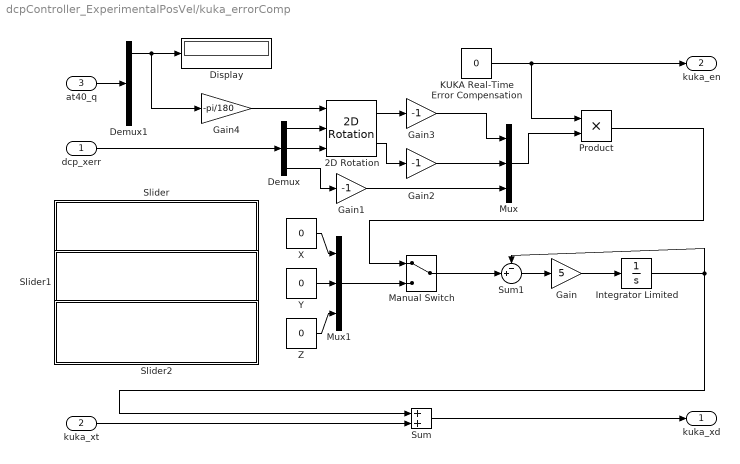
== system dcpController_ExperimentalPosVel/kuka_errorComp ==
  dcp_xerr : Inport
  "kuka_xt " : Inport  Port=2
  at40_q : Inport  Port=3
  2D Rotation : dcpctrl/2D Rotation
  Demux : Demux  Outputs=3
  Demux1 : Demux
  Display : Display
  Gain : Gain  Gain=5
  Gain1 : Gain  Gain=-1
  Gain2 : Gain  Gain=-1
  Gain3 : Gain  Gain=-1
  Gain4 : Gain  Gain=-pi/180
  Integrator Limited : Integrator  LimitOutput=on  UpperSaturationLimit=100  LowerSaturationLimit=-100
  KUKA Real-Time Error Compensation : Constant  Value=0
  Manual Switch : ManualSwitch
  Mux : Mux  Inputs=3
  Mux1 : Mux  Inputs=3
  Product : Product
  Slider : Subsystem  DialogController=hmiCreateDDGDialog  IsWebBlock=on  mask(MWDashboardBlock){webBlockId=caea66fb-15d0-453b-a290-cafa8ad2d763, webBlockType=slider, ShowInLibBrowser=on, ShowInitialText=on, HMISrcModelName=dcpController_ExperimentalPosVel}
      mask prompts: webBlockId "WebBlock Id"; webBlockType "WebBlock Type"; HMISrcModelName "Source Model"
      mask help: SimulinkHMI:dialogs:SliderDialogDesc
      mask Help: helpview([docroot '/mapfiles/simulink.map'], 'hmi_slider')
      mask Display:
      | if strcmp(get_param(bdroot(gcb),'BlockDiagramType'), 'library')
      |     image([(matlabroot) '/toolbox/simulink/hmi/icons/Slider.png']);
      | end
  Slider1 : Subsystem  DialogController=hmiCreateDDGDialog  IsWebBlock=on  mask(MWDashboardBlock){webBlockId=c5c2bbba-e352-4fbf-87a3-2c33520b8894, webBlockType=slider, ShowInLibBrowser=on, ShowInitialText=on, HMISrcModelName=dcpController_ExperimentalPosVel}
      mask prompts: webBlockId "WebBlock Id"; webBlockType "WebBlock Type"; HMISrcModelName "Source Model"
      mask help: SimulinkHMI:dialogs:SliderDialogDesc
      mask Help: helpview([docroot '/mapfiles/simulink.map'], 'hmi_slider')
      mask Display:
      | if strcmp(get_param(bdroot(gcb),'BlockDiagramType'), 'library')
      |     image([(matlabroot) '/toolbox/simulink/hmi/icons/Slider.png']);
      | end
  Slider2 : Subsystem  DialogController=hmiCreateDDGDialog  IsWebBlock=on  mask(MWDashboardBlock){webBlockId=3919ddfc-a7e7-401f-81de-b7753522eb96, webBlockType=slider, ShowInLibBrowser=on, ShowInitialText=on, HMISrcModelName=dcpController_ExperimentalPosVel}
      mask prompts: webBlockId "WebBlock Id"; webBlockType "WebBlock Type"; HMISrcModelName "Source Model"
      mask help: SimulinkHMI:dialogs:SliderDialogDesc
      mask Help: helpview([docroot '/mapfiles/simulink.map'], 'hmi_slider')
      mask Display:
      | if strcmp(get_param(bdroot(gcb),'BlockDiagramType'), 'library')
      |     image([(matlabroot) '/toolbox/simulink/hmi/icons/Slider.png']);
      | end
  Sum : Sum
  Sum1 : Sum  Inputs=-+|
  X : Constant  Value=0
  Y : Constant  Value=0
  Z : Constant  Value=0
  kuka_xd : Outport
  kuka_en : Outport  Port=2
  wires:
  "kuka_xt "/1 -> Sum/2
  Demux/1 -> 2D Rotation/2
  Demux/2 -> 2D Rotation/3
  2D Rotation/1 -> Gain3/1
  2D Rotation/2 -> Gain2/1
  Demux/3 -> Gain1/1
  Mux1/1 -> Manual Switch/2
  at40_q/1 -> Demux1/1
  Demux1/1 -> Display/1, Gain4/1
  Mux/1 -> Product/2
  KUKA Real-Time Error Compensation/1 -> kuka_en/1, Product/1
  Gain/1 -> Integrator Limited/1
  Gain1/1 -> Mux/3
  Gain2/1 -> Mux/2
  Gain3/1 -> Mux/1
  Integrator Limited/1 -> Sum1/1, Sum/1
  X/1 -> Mux1/1
  Z/1 -> Mux1/3
  Sum/1 -> kuka_xd/1
  Product/1 -> Manual Switch/1
  Manual Switch/1 -> Sum1/2
  Sum1/1 -> Gain/1
  Y/1 -> Mux1/2
  Gain4/1 -> 2D Rotation/1
  dcp_xerr/1 -> Demux/1

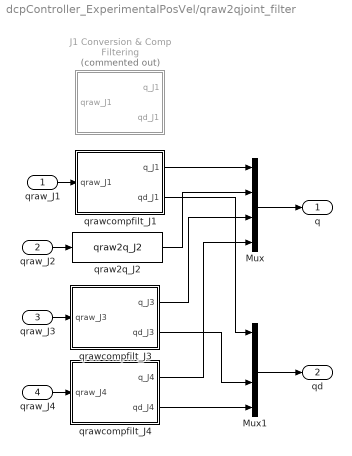
== system dcpController_ExperimentalPosVel/qraw2qjoint_filter ==
  qraw_J1 : Inport
  qraw_J2 : Inport  Port=2
  qraw_J3 : Inport  Port=3
  qraw_J4 : Inport  Port=4
  J1 Conversion & Comp Filtering : Subsystem  Commented=on
  Mux : Mux
  Mux1 : Mux
  qraw2q_J2 : dcpctrl/qraw2q_J2
  qrawcompfilt_J1 : Subsystem
  qrawcompfilt_J3 : Subsystem
  qrawcompfilt_J4 : Subsystem
  q : Outport
  qd : Outport  Port=2
  wires:
  qraw_J2/1 -> qraw2q_J2/1
  qraw_J1/1 -> qrawcompfilt_J1/1(qraw_J1)
  qraw_J4/1 -> qrawcompfilt_J4/1(qraw_J4)
  qraw_J3/1 -> qrawcompfilt_J3/1(qraw_J3)
  qrawcompfilt_J4/2(qd_J4) -> Mux1/4
  qrawcompfilt_J3/2(qd_J3) -> Mux1/3
  qrawcompfilt_J1/2(qd_J1) -> Mux1/1
  qrawcompfilt_J1/1(q_J1) -> Mux/1
  qraw2q_J2/1 -> Mux/2
  qrawcompfilt_J3/1(q_J3) -> Mux/3
  qrawcompfilt_J4/1(q_J4) -> Mux/4
  Mux1/1 -> qd/1
  Mux/1 -> q/1

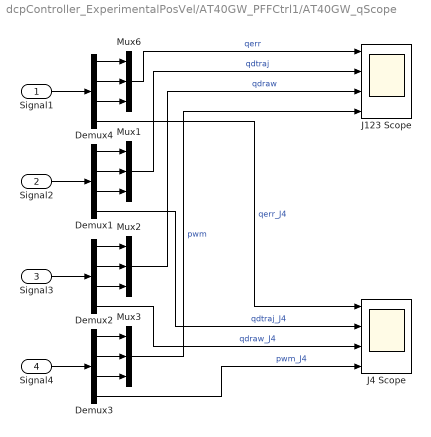
== system dcpController_ExperimentalPosVel/AT40GW_PFFCtrl1/AT40GW_qScope ==
  Signal1 : Inport
  Signal2 : Inport  Port=2
  Signal3 : Inport  Port=3
  Signal4 : Inport  Port=4
  Demux{1..4} (4 alike) : Demux
  J123 Scope : Scope  NumInputPorts=4
  J4 Scope : Scope  NumInputPorts=4
  Mux{1..3,6} (4 alike) : Mux  Inputs=3
  wires:
  Demux4/1 -> Mux6/1
  Demux2/1 -> Mux2/1
  Demux3/4 -> J4 Scope/4  "pwm_J4"
  Demux4/4 -> J4 Scope/1  "qerr_J4"
  Mux2/1 -> J123 Scope/3  "qdraw"
  Mux1/1 -> J123 Scope/2  "qdtraj"
  Demux3/3 -> Mux3/3
  Demux3/2 -> Mux3/2
  Signal4/1 -> Demux3/1
  Demux3/1 -> Mux3/1
  Demux2/3 -> Mux2/3
  Demux2/2 -> Mux2/2
  Signal3/1 -> Demux2/1
  Demux1/3 -> Mux1/3
  Demux1/2 -> Mux1/2
  Signal2/1 -> Demux1/1
  Demux1/1 -> Mux1/1
  Demux4/3 -> Mux6/3
  Demux4/2 -> Mux6/2
  Signal1/1 -> Demux4/1
  Mux6/1 -> J123 Scope/1  "qerr"
  Demux1/4 -> J4 Scope/2  "qdtraj_J4"
  Demux2/4 -> J4 Scope/3  "qdraw_J4"
  Mux3/1 -> J123 Scope/4  "pwm"

== system dcpController_ExperimentalPosVel/AT40GW_PFFCtrl1/FF 10^n Gain Adjustment ==
  Constant : Constant
  FF Gain : Gain  Gain=[1,1,1,1]
  GainAdj_J1FF : Constant  Value=-1.108333333333333
  GainAdj_J2FF : Constant  Value=0
  GainAdj_J3FF : Constant  Value=-0.7083333333333333
  GainAdj_J4FF : Constant  Value=-0.4583333333333335
  Math Function{,1..3} (4 alike) : Math  Operator=10^u  SaturateOnIntegerOverflow=on
  Mux1 : Mux
  Product : Product
  Out1 : Outport
  wires:
  FF Gain/1 -> Product/2
  Constant/1 -> FF Gain/1
  GainAdj_J4FF/1 -> Math Function3/1
  GainAdj_J3FF/1 -> Math Function2/1
  GainAdj_J2FF/1 -> Math Function1/1
  GainAdj_J1FF/1 -> Math Function/1
  Math Function2/1 -> Mux1/3
  Math Function3/1 -> Mux1/4
  Mux1/1 -> Product/1, Out1/1
  Math Function/1 -> Mux1/1
  Math Function1/1 -> Mux1/2

== system dcpController_ExperimentalPosVel/AT40GW_PFFCtrl1/P 10^n Gain Adjustment ==
  Constant : Constant
  GainAdj_J1 : Constant  Value=-0.3
  GainAdj_J2 : Constant
  GainAdj_J3 : Constant  Value=-0.266666666667
  GainAdj_J4 : Constant  Value=-0.583333333333
  Math Function{,1..3} (4 alike) : Math  Operator=10^u  SaturateOnIntegerOverflow=on
  Mux1 : Mux
  P Gain : Gain  Gain=[robot.Joint(:).Kp]
  Product : Product
  Out1 : Outport
  wires:
  P Gain/1 -> Product/2
  Constant/1 -> P Gain/1
  GainAdj_J4/1 -> Math Function3/1
  GainAdj_J3/1 -> Math Function2/1
  GainAdj_J2/1 -> Math Function1/1
  GainAdj_J1/1 -> Math Function/1
  Math Function2/1 -> Mux1/3
  Math Function3/1 -> Mux1/4
  Mux1/1 -> Product/1, Out1/1
  Math Function/1 -> Mux1/1
  Math Function1/1 -> Mux1/2

== system dcpController_ExperimentalPosVel/AT40GW_PFFCtrl1/qd2qdraw ==
  q : Inport
  qd : Inport  Port=2
  dj2drfcn : MATLAB Function  TreatAsAtomicUnit=on
  qdraw : Outport
  wires:
  q/1 -> dj2drfcn/1(q)
  dj2drfcn/1(qdraw) -> qdraw/1
  qd/1 -> dj2drfcn/2(qd)

== system dcpController_ExperimentalPosVel/AT40GW_PFFCtrl1/qdraw2pwm ==
  qdraw : Inport
  Demux : Demux
  Mux : Mux
  qdraw2pwm_J1 : Subsystem
  qdraw2pwm_J2 : Subsystem
  qdraw2pwm_J3 : Subsystem
  qdraw2pwm_J4 : Subsystem
  pwm : Outport
  wires:
  qdraw2pwm_J1/1(pwm_J1) -> Mux/1
  qdraw2pwm_J2/1(pwm_J2) -> Mux/2
  Mux/1 -> pwm/1
  qdraw2pwm_J3/1(pwm_J3) -> Mux/3
  qdraw2pwm_J4/1(pwm_J4) -> Mux/4
  Demux/4 -> qdraw2pwm_J4/1(qdraw_J4)
  Demux/2 -> qdraw2pwm_J2/1(qdraw_J2)
  Demux/3 -> qdraw2pwm_J3/1(qdraw_J3)
  Demux/1 -> qdraw2pwm_J1/1(qdraw_J1)
  qdraw/1 -> Demux/1

== system dcpController_ExperimentalPosVel/AT40GW_PosVelCtrl/q_I 10^n Gain Adjustment ==
  GainAdj_J1qI : Constant  Value=-1.941176470588
  GainAdj_J2qI : Constant  Value=0
  GainAdj_J3qI : Constant  Value=-1.788235294118
  GainAdj_J4qI : Constant  Value=-1.623529411765
  Math Function{,1..3} (4 alike) : Math  Operator=10^u  SaturateOnIntegerOverflow=on
  Mux1 : Mux
  Out1 : Outport
  wires:
  Math Function1/1 -> Mux1/2
  Math Function/1 -> Mux1/1
  Mux1/1 -> Out1/1
  Math Function3/1 -> Mux1/4
  Math Function2/1 -> Mux1/3
  GainAdj_J1qI/1 -> Math Function/1
  GainAdj_J2qI/1 -> Math Function1/1
  GainAdj_J3qI/1 -> Math Function2/1
  GainAdj_J4qI/1 -> Math Function3/1

== system dcpController_ExperimentalPosVel/AT40GW_PosVelCtrl/q_P 10^n Gain Adjustment ==
  GainAdj_J1qP : Constant  Value=0.2154696132597
  GainAdj_J2qP : Constant  Value=0
  GainAdj_J3qP : Constant  Value=-0.187845303867
  GainAdj_J4qP : Constant  Value=-0.491712707182
  Math Function : Math  Operator=10^u  SaturateOnIntegerOverflow=on
  Math Function2 : Math  Operator=10^u  SaturateOnIntegerOverflow=on
  Math Function3 : Math  Operator=10^u  SaturateOnIntegerOverflow=on
  Mux1 : Mux
  Out1 : Outport
  wires:
  GainAdj_J2qP/1 -> Mux1/2
  Math Function/1 -> Mux1/1
  Mux1/1 -> Out1/1
  Math Function3/1 -> Mux1/4
  Math Function2/1 -> Mux1/3
  GainAdj_J1qP/1 -> Math Function/1
  GainAdj_J3qP/1 -> Math Function2/1
  GainAdj_J4qP/1 -> Math Function3/1

== system dcpController_ExperimentalPosVel/AT40GW_PosVelCtrl/qd_FF 10^n Gain Adjustment ==
  GainAdj_J1qdFF : Constant  Value=-0.018382352941
  GainAdj_J2qdFF : Constant  Value=0
  GainAdj_J3qdFF : Constant  Value=-0.0625
  GainAdj_J4qd FF : Constant  Value=-0.002259036145
  Math Function{,1..3} (4 alike) : Math  Operator=10^u  SaturateOnIntegerOverflow=on
  Mux1 : Mux
  Out1 : Outport
  wires:
  GainAdj_J4qd FF/1 -> Math Function3/1
  GainAdj_J3qdFF/1 -> Math Function2/1
  GainAdj_J2qdFF/1 -> Math Function1/1
  GainAdj_J1qdFF/1 -> Math Function/1
  Math Function2/1 -> Mux1/3
  Math Function3/1 -> Mux1/4
  Mux1/1 -> Out1/1
  Math Function/1 -> Mux1/1
  Math Function1/1 -> Mux1/2

== system dcpController_ExperimentalPosVel/AT40GW_PosVelCtrl/qd_I 10^n Gain Adjustment ==
  GainAdj_J1qdI : Constant  Value=-1.188235294118
  GainAdj_J2qdI : Constant  Value=0
  GainAdj_J3qdI : Constant  Value=-0.941176470588
  GainAdj_J4qdI : Constant  Value=-2.552941176471
  Math Function{,1..3} (4 alike) : Math  Operator=10^u  SaturateOnIntegerOverflow=on
  Mux1 : Mux
  Out1 : Outport
  wires:
  Math Function1/1 -> Mux1/2
  Math Function/1 -> Mux1/1
  Mux1/1 -> Out1/1
  Math Function3/1 -> Mux1/4
  Math Function2/1 -> Mux1/3
  GainAdj_J1qdI/1 -> Math Function/1
  GainAdj_J2qdI/1 -> Math Function1/1
  GainAdj_J3qdI/1 -> Math Function2/1
  GainAdj_J4qdI/1 -> Math Function3/1

== system dcpController_ExperimentalPosVel/AT40GW_PosVelCtrl/qd_P 10^n Gain Adjustment ==
  GainAdj_J1qdP : Constant  Value=-2.082352941176
  GainAdj_J2qdP : Constant
  GainAdj_J3qdP : Constant  Value=-2
  GainAdj_J4qdP : Constant  Value=-3.4
  Math Function{,1..3} (4 alike) : Math  Operator=10^u  SaturateOnIntegerOverflow=on
  Mux1 : Mux
  Out1 : Outport
  wires:
  GainAdj_J4qdP/1 -> Math Function3/1
  GainAdj_J3qdP/1 -> Math Function2/1
  GainAdj_J2qdP/1 -> Math Function1/1
  GainAdj_J1qdP/1 -> Math Function/1
  Math Function2/1 -> Mux1/3
  Math Function3/1 -> Mux1/4
  Mux1/1 -> Out1/1
  Math Function/1 -> Mux1/1
  Math Function1/1 -> Mux1/2

== system dcpController_ExperimentalPosVel/AT40GW_qqdCtrl1/q_P 10^n Gain Adjustment ==
  GainAdj_J1qP : Constant  Value=0.5157894736842
  GainAdj_J2qP : Constant  Value=0
  GainAdj_J3qP : Constant  Value=0.8
  GainAdj_J4qP : Constant  Value=0.936170212766
  Math Function : Math  Operator=10^u  SaturateOnIntegerOverflow=on
  Math Function2 : Math  Operator=10^u  SaturateOnIntegerOverflow=on
  Math Function3 : Math  Operator=10^u  SaturateOnIntegerOverflow=on
  Mux1 : Mux
  Out1 : Outport
  wires:
  GainAdj_J2qP/1 -> Mux1/2
  Math Function/1 -> Mux1/1
  Mux1/1 -> Out1/1
  Math Function3/1 -> Mux1/4
  Math Function2/1 -> Mux1/3
  GainAdj_J1qP/1 -> Math Function/1
  GainAdj_J3qP/1 -> Math Function2/1
  GainAdj_J4qP/1 -> Math Function3/1

== system dcpController_ExperimentalPosVel/AT40GW_qqdCtrl1/qd_FF 10^n Gain Adjustment ==
  GainAdj_J1qdFF : Constant  Value=-1.815642458101
  GainAdj_J2qdFF : Constant  Value=0
  GainAdj_J3qdFF : Constant  Value=-1.391061452514
  GainAdj_J4qd FF : Constant  Value=-2.865921787709
  Math Function{,1..3} (4 alike) : Math  Operator=10^u  SaturateOnIntegerOverflow=on
  Mux1 : Mux
  Out1 : Outport
  wires:
  GainAdj_J4qd FF/1 -> Math Function3/1
  GainAdj_J3qdFF/1 -> Math Function2/1
  GainAdj_J2qdFF/1 -> Math Function1/1
  GainAdj_J1qdFF/1 -> Math Function/1
  Math Function2/1 -> Mux1/3
  Math Function3/1 -> Mux1/4
  Mux1/1 -> Out1/1
  Math Function/1 -> Mux1/1
  Math Function1/1 -> Mux1/2

== system dcpController_ExperimentalPosVel/AT40GW_qqdCtrl1/qd_P 10^n Gain Adjustment ==
  GainAdj_J1qdP : Constant  Value=-1.648044692737
  GainAdj_J2qdP : Constant
  GainAdj_J3qdP : Constant  Value=-1.849162011173
  GainAdj_J4qdP : Constant  Value=-3.128491620112
  Math Function{,1..3} (4 alike) : Math  Operator=10^u  SaturateOnIntegerOverflow=on
  Mux1 : Mux
  Out1 : Outport
  wires:
  GainAdj_J4qdP/1 -> Math Function3/1
  GainAdj_J3qdP/1 -> Math Function2/1
  GainAdj_J2qdP/1 -> Math Function1/1
  GainAdj_J1qdP/1 -> Math Function/1
  Math Function2/1 -> Mux1/3
  Math Function3/1 -> Mux1/4
  Mux1/1 -> Out1/1
  Math Function/1 -> Mux1/1
  Math Function1/1 -> Mux1/2

== system dcpController_ExperimentalPosVel/Control Panel/Push Button ==

== system dcpController_ExperimentalPosVel/Control Panel/Slider Switch ==

== system dcpController_ExperimentalPosVel/Control Panel/Slider7 ==

== system dcpController_ExperimentalPosVel/Gain Tuning/Slider1 ==

== system dcpController_ExperimentalPosVel/Gain Tuning/Slider12 ==

== system dcpController_ExperimentalPosVel/Gain Tuning/Slider13 ==

== system dcpController_ExperimentalPosVel/Gain Tuning/Slider14 ==

== system dcpController_ExperimentalPosVel/Gain Tuning/Slider15 ==

== system dcpController_ExperimentalPosVel/Gain Tuning/Slider16 ==

== system dcpController_ExperimentalPosVel/Gain Tuning/Slider17 ==

== system dcpController_ExperimentalPosVel/Gain Tuning/Slider18 ==

== system dcpController_ExperimentalPosVel/Gain Tuning/Slider2 ==

== system dcpController_ExperimentalPosVel/Gain Tuning/Slider3 ==

== system dcpController_ExperimentalPosVel/Gain Tuning/Slider4 ==

== system dcpController_ExperimentalPosVel/Gain Tuning/Slider5 ==

== system dcpController_ExperimentalPosVel/Gain Tuning/Slider6 ==

== system dcpController_ExperimentalPosVel/Gain Tuning/Slider8 ==

== system dcpController_ExperimentalPosVel/Gain Tuning/Slider9 ==

== system dcpController_ExperimentalPosVel/kuka_errorComp/Slider ==

== system dcpController_ExperimentalPosVel/kuka_errorComp/Slider1 ==

== system dcpController_ExperimentalPosVel/kuka_errorComp/Slider2 ==

== system dcpController_ExperimentalPosVel/qraw2qjoint_filter/J1 Conversion & Comp Filtering ==
  qraw_J1 : Inport
  Complementary Filter : dcpctrl/complementaryFilter
  DCP Scope : Scope
  Demux1 : Demux  Outputs=2
  Equal Moving Average : DiscreteFir  Coefficients=[0.1 0.1 0.1 0.1 0.1 0.1 0.1 0.1 0.1 0.1]  InputProcessing=Columns as channels (frame based)
  Mux1 : Mux  Inputs=3
  Slider : Subsystem  DialogController=hmiCreateDDGDialog  IsWebBlock=on  mask(MWDashboardBlock){webBlockId=6cb21987-2b01-4c45-884a-14f8bf8cd4b2, webBlockType=slider, ShowInLibBrowser=on, ShowInitialText=on, HMISrcModelName=dcpController_ExperimentalPosVel}
      mask prompts: webBlockId "WebBlock Id"; webBlockType "WebBlock Type"; HMISrcModelName "Source Model"
      mask help: SimulinkHMI:dialogs:SliderDialogDesc
      mask Help: helpview([docroot '/mapfiles/simulink.map'], 'hmi_slider')
      mask Display:
      | if strcmp(get_param(bdroot(gcb),'BlockDiagramType'), 'library')
      |     image([(matlabroot) '/toolbox/simulink/hmi/icons/Slider.png']);
      | end
  compFiltTau_J1 : Constant  Value=0.5
  qraw2q_J1 : dcpctrl/qraw2q_J1
  q_J1 : Outport
  qd_J1 : Outport  Port=2
  wires:
  Equal Moving Average/1 -> qd_J1/1
  qraw_J1/1 -> qraw2q_J1/1
  Demux1/2 -> Complementary Filter/2, Mux1/1
  Demux1/1 -> Mux1/2
  compFiltTau_J1/1 -> Complementary Filter/3
  qraw2q_J1/1 -> Demux1/1
  qraw2q_J1/2 -> Equal Moving Average/1, Complementary Filter/1
  Complementary Filter/1 -> q_J1/1, Mux1/3
  Mux1/1 -> DCP Scope/1

== system dcpController_ExperimentalPosVel/qraw2qjoint_filter/qrawcompfilt_J1 ==
  note: NOTE: This function still requires refinement after the J1 absolute sensor is installed. Tasks include:
      | - Replacing complementary filter (or other appropriate filtering)
      | - Re-enabling J1 absolute input (removing J1 Absolute Reference block)
  qraw_J1 : Inport
  Demux : Demux  Outputs=2
  Demux1 : Demux  Outputs=2
  Equal Moving Average : DiscreteFir  Coefficients=repmat([1/50],1,50)  InputProcessing=Columns as channels (frame based)
  J1 Absolute Reference : Constant  Value=5
  Mux : Mux  Inputs=2
  qraw2q_J1 : dcpctrl/qraw2q_J1
  q_J1 : Outport
  qd_J1 : Outport  Port=2
  wires:
  qraw2q_J1/1 -> Demux1/1
  qraw2q_J1/2 -> Equal Moving Average/1
  Equal Moving Average/1 -> qd_J1/1
  Demux1/1 -> q_J1/1
  qraw_J1/1 -> Demux/1
  Demux/1 -> Mux/1
  Mux/1 -> qraw2q_J1/1
  Demux/2 -> Mux/2
